simulink model "ContinuousDCMotorSimulation"  (R2018b)
settings: Solver=VariableStepAuto  StartTime=0.0  StopTime=Tf  MaxStep=Ts  RelTol=1e-3
values from neighbouring files (symbols this model uses):
  C0 = 0.0    (= 0)    [DCMotorParameters.m]
  F = 0.0001    [DCMotorParameters.m]
  Imax = Inom    (= 5)    [DCMotorParameters.m]
  Imin = -Inom    (= -5)    [DCMotorParameters.m]
  J = 2.20e-4    (= 0.00022)    [DCMotorParameters.m]
  Ke = place(Ae,Be,Elec_desired_poles)    [DCMotorParameters.m]
  Km = place(Am,Bm,Desired_mecha_pole)    [DCMotorParameters.m]
  Kphi = 0.061    [DCMotorParameters.m]
  L = 2.7e-3    (= 0.0027)    [DCMotorParameters.m]
  R = 1.22    [DCMotorParameters.m]
  Vmax = Vdc    (= 24)    [DCMotorParameters.m]
  Vmin = -Vdc    (= -24)    [DCMotorParameters.m]
libraries: simulink x4
Description:
  | Continuous time model of the DC motor
  | 
  | Cascaded speed control :
  | - Inner loop : electrical control (state feedback with integral action)
  | - Outer loop :  mechanical control (state feedback with integral action)
  | - Clamping : Enable or disable integral actions
settings Model: Creator=R.Delpoux & L.Kerhuel  LastModifiedBy=rdelpoux
settings SolverCC: ZeroCrossControl=DisableAll
settings SFSimCC: SimUseLocalCustomCode=off
settings RTWCC: RTWUseLocalCustomCode=off

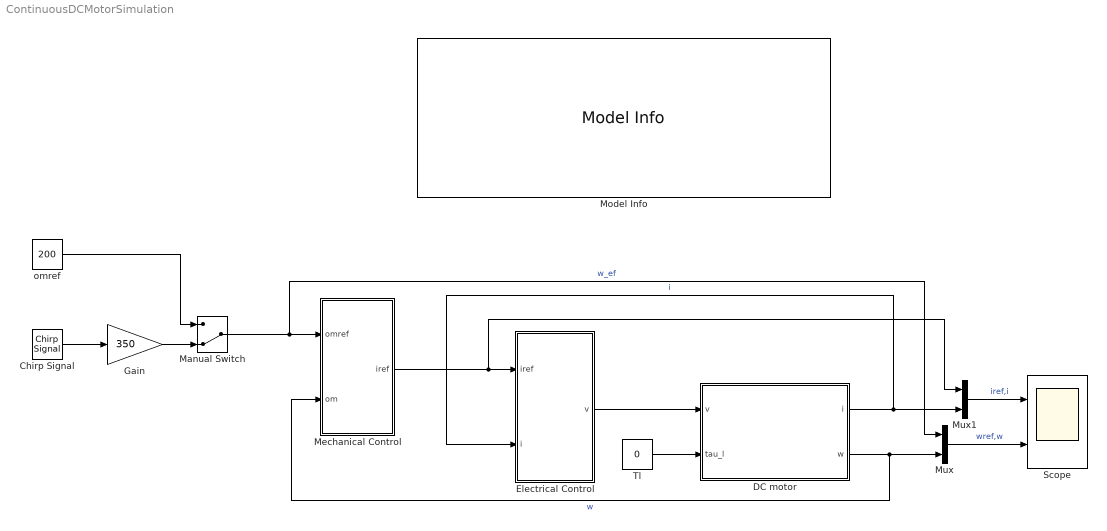
== system ContinuousDCMotorSimulation ==
  Chirp Signal : simulink/Sources/Chirp Signal  f1=0.1  T=20  f2=5
  DC motor : Subsystem  mask(Motor PRAVALUX MPM4-0002){R=R, L=L, Kphi=Kphi, J=J, F=F, C0=C0}
      mask prompts: R "Resistance (R) in Ohms"; L "Inductance (L) in H"; Kphi "Back EMF (Kphi) in V/rad/s"; J "J in kgm²"; F "F in N/rad/s"
      mask help:
      | Continuous time Model for PRAVALUX MPM4 DC motor
      | Caracteristics: 24V DC, 90W, 5.2A, 3000RPM
      |
      | It is a 2nd order model made of two intertwinned system:
      | one 1st order electrical system and one 1st order mechanical system.
      |
      | Look under mask (Ctrl-U) to see the model
      mask DialogControl Container11 Prompt: Motor
      mask DialogControl Container3 Prompt: Electrical Parameters
      mask DialogControl Container3_copy Prompt: Mechanical Parameters
      mask Display:
      | color('green');
      | image('MotorPravalux.png');
      | %port_label('input',1,'DC');
      | %port_label('output',1,'BEMF');
  Electrical Control : Subsystem
  Gain : Gain  Gain=350  OutDataTypeStr=Inherit: Inherit via back propagation
  Manual Switch : ManualSwitch  CurrentSetting=0
  Mechanical Control : Subsystem
  Model Info : simulink/Model-Wide Utilities/Model Info  Frame=on  DisplayStringWithTags=|  HorizontalTextAlignment=Center  LeftAlignmentValue=0.5
      | %<ModelName> v%<ModelVersion> - %<Creator>
      | 
      | %<Description>
      | 
      | Lost modified on: %<LastModificationDate>
  Mux : Mux  Inputs=2
  Mux1 : Mux  Inputs=2
  Scope : Scope  NumInputPorts=2
  Tl : Constant  Value=0
  omref : Constant  Value=200  OutDataTypeStr=Inherit: Inherit via back propagation
  wires:
  Electrical Control/1(v) -> DC motor/1(v)
  DC motor/2(w) -> Mux/2, Mechanical Control/2(om)  "w"
  DC motor/1(i) -> Electrical Control/2(i), Mux1/2  "i"
  Mux/1 -> Scope/2  "wref,w"
  Manual Switch/1 -> Mechanical Control/1(omref), Mux/1  "w_ef"
  Mux1/1 -> Scope/1  "iref,i"
  Mechanical Control/1(iref) -> Mux1/1, Electrical Control/1(iref)
  Tl/1 -> DC motor/2(tau_l)
  Gain/1 -> Manual Switch/2
  Chirp Signal/1 -> Gain/1
  omref/1 -> Manual Switch/1

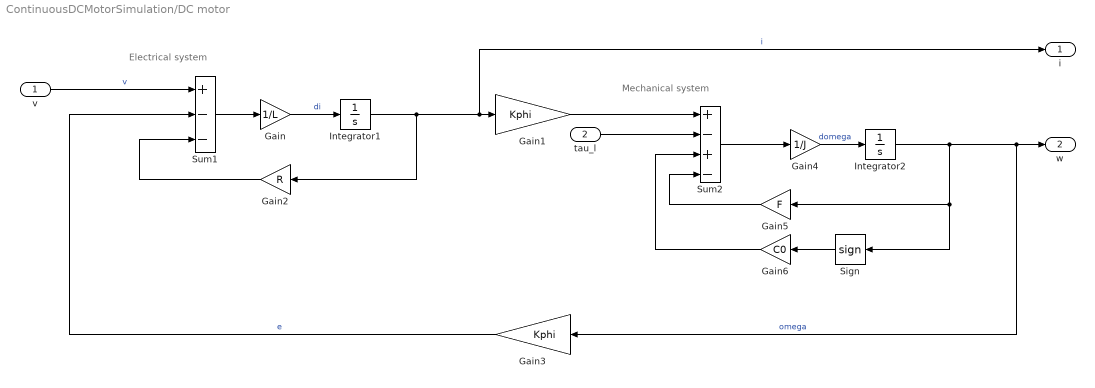
== system ContinuousDCMotorSimulation/DC motor ==
  note: Mechanical system
  note: Electrical system
  v : Inport  SampleTime=0
  tau_l : Inport  Port=2
  Gain : Gain  Gain=1/L
  Gain1 : Gain  Gain=Kphi
  Gain2 : Gain  Gain=R
  "Gain3  " : Gain  Gain=Kphi
  Gain4 : Gain  Gain=1/J
  Gain5 : Gain  Gain=F
  Gain6 : Gain  Gain=C0
  Integrator1 : Integrator
  Integrator2 : Integrator
  Sign : Signum
  Sum1 : Sum  Inputs=+--
  Sum2 : Sum  Inputs=+-+-
  i : Outport
  w : Outport  Port=2
  wires:
  Sum1/1 -> Gain/1
  Gain/1 -> Integrator1/1  "di"
  Integrator1/1 -> Gain2/1, i/1, Gain1/1  "i"
  v/1 -> Sum1/1  "v"
  Gain2/1 -> Sum1/3
  "Gain3  "/1 -> Sum1/2  "e"
  tau_l/1 -> Sum2/2
  Gain6/1 -> Sum2/3
  Sign/1 -> Gain6/1
  Integrator2/1 -> "Gain3  "/1, w/1, Sign/1, Gain5/1  "omega"
  Gain5/1 -> Sum2/4
  Sum2/1 -> Gain4/1
  Gain4/1 -> Integrator2/1  "domega"
  Gain1/1 -> Sum2/1

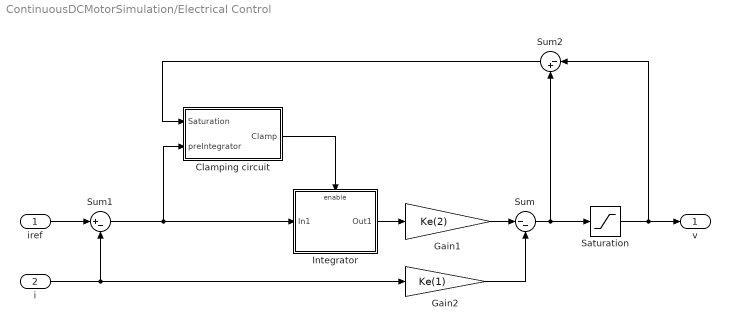
== system ContinuousDCMotorSimulation/Electrical Control ==
  iref : Inport
  i : Inport  Port=2
  Clamping circuit : Subsystem
  Gain1 : Gain  Gain=Ke(2)
  Gain2 : Gain  Gain=Ke(1)
  Integrator : Subsystem
  Saturation : Saturate  UpperLimit=Vmax  LowerLimit=Vmin
  Sum : Sum  Inputs=|--
  Sum1 : Sum  Inputs=|+-
  Sum2 : Sum  Inputs=|-+  OutDataTypeStr=Inherit: Same as accumulator
  v : Outport
  wires:
  iref/1 -> Sum1/1
  i/1 -> Gain2/1, Sum1/2
  Gain1/1 -> Sum/1
  Gain2/1 -> Sum/2
  Saturation/1 -> Sum2/1, v/1
  Sum1/1 -> Integrator/1(In1), Clamping circuit/2(preIntegrator)
  Integrator/1(Out1) -> Gain1/1
  Clamping circuit/1(Clamp) -> Integrator/Enable
  Sum/1 -> Saturation/1, Sum2/2
  Sum2/1 -> Clamping circuit/1(Saturation)

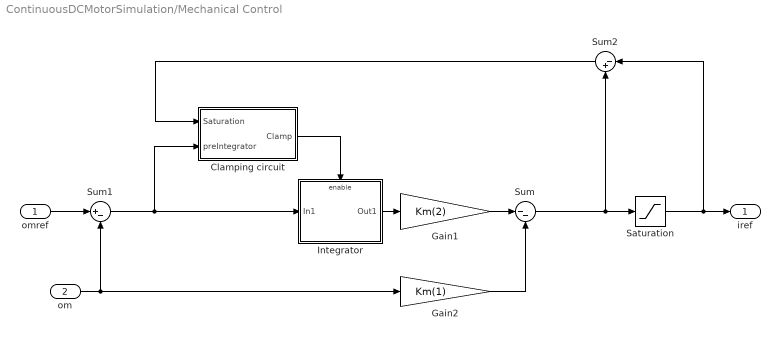
== system ContinuousDCMotorSimulation/Mechanical Control ==
  omref : Inport
  om : Inport  Port=2
  Clamping circuit : Subsystem
  Gain1 : Gain  Gain=Km(2)
  Gain2 : Gain  Gain=Km(1)
  Integrator : Subsystem
  Saturation : Saturate  UpperLimit=Imax  LowerLimit=Imin
  Sum : Sum  Inputs=|--
  Sum1 : Sum  Inputs=|+-
  Sum2 : Sum  Inputs=|-+  OutDataTypeStr=Inherit: Same as accumulator
  iref : Outport
  wires:
  Gain1/1 -> Sum/1
  Sum1/1 -> Clamping circuit/2(preIntegrator), Integrator/1(In1)
  omref/1 -> Sum1/1
  Gain2/1 -> Sum/2
  om/1 -> Gain2/1, Sum1/2
  Sum2/1 -> Clamping circuit/1(Saturation)
  Sum/1 -> Sum2/2, Saturation/1
  Clamping circuit/1(Clamp) -> Integrator/Enable
  Saturation/1 -> Sum2/1, iref/1
  Integrator/1(Out1) -> Gain1/1

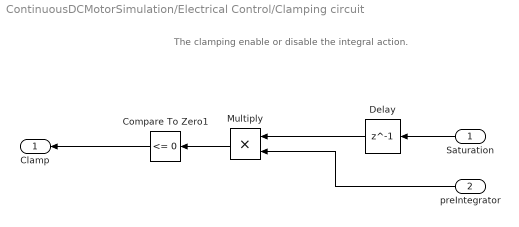
== system ContinuousDCMotorSimulation/Electrical Control/Clamping circuit ==
  note: The clamping enable or disable the integral action.
  Saturation : Inport  DisableCoverage=on
  preIntegrator : Inport  DisableCoverage=on  Port=2
  Compare To Zero1 : simulink/Logic and Bit Operations/Compare To Zero  relop=<=  OutDataTypeStr=boolean
  Delay : Delay  DelayLength=1  InitialCondition=0
  Multiply : Product
  Clamp : Outport  DisableCoverage=on
  wires:
  Compare To Zero1/1 -> Clamp/1
  preIntegrator/1 -> Multiply/2
  Multiply/1 -> Compare To Zero1/1
  Saturation/1 -> Delay/1
  Delay/1 -> Multiply/1

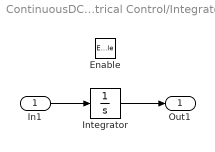
== system ContinuousDCMotorSimulation/Electrical Control/Integrator ==
  In1 : Inport
  Enable : EnablePort
  Integrator : Integrator
  Out1 : Outport
  wires:
  Integrator/1 -> Out1/1
  In1/1 -> Integrator/1

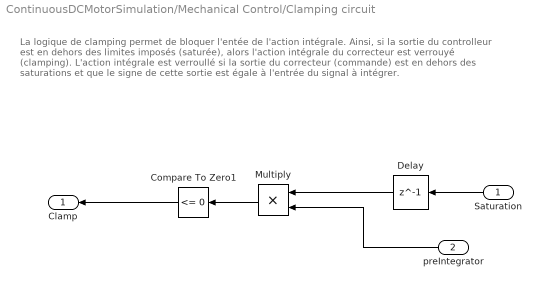
== system ContinuousDCMotorSimulation/Mechanical Control/Clamping circuit ==
  note: La logique de clamping permet de bloquer l'entée de l'action intégrale.
      | Ainsi, si la sortie du controlleur est en dehors des limites imposés (saturée), alors l'action intégrale du correcteur est verrouyé (clamping).
      | L'action intégrale est verroullé si la sortie du correcteur (commande) est en dehors des saturations et que le signe de cette sortie est égale
      | à l'entrée du signal à intégrer.
  Saturation : Inport  DisableCoverage=on
  preIntegrator : Inport  DisableCoverage=on  Port=2
  Compare To Zero1 : simulink/Logic and Bit Operations/Compare To Zero  relop=<=  OutDataTypeStr=boolean
  Delay : Delay  DelayLength=1  InitialCondition=0
  Multiply : Product
  Clamp : Outport  DisableCoverage=on
  wires:
  Compare To Zero1/1 -> Clamp/1
  preIntegrator/1 -> Multiply/2
  Multiply/1 -> Compare To Zero1/1
  Saturation/1 -> Delay/1
  Delay/1 -> Multiply/1

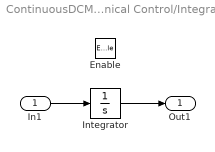
== system ContinuousDCMotorSimulation/Mechanical Control/Integrator ==
  In1 : Inport
  Enable : EnablePort
  Integrator : Integrator
  Out1 : Outport
  wires:
  Integrator/1 -> Out1/1
  In1/1 -> Integrator/1
